simulink model "Controlled_SinglePhase_CenterTapde_Rectifier"  (R2021a)
settings: Solver=VariableStepAuto  StartTime=0.0  StopTime=0.1  MaxStep=1e-6  RelTol=1e-3
libraries: spsGroundLib x2, spsThyristorLib x2, spsVoltageMeasurementLib x2, spsACVoltageSourceLib x1, spsLinearTransformerLib x1, spsSeriesRLCBranchLib x1, spspowerguiLib x1
settings Model: Creator=mluser  LastModifiedBy=mluser

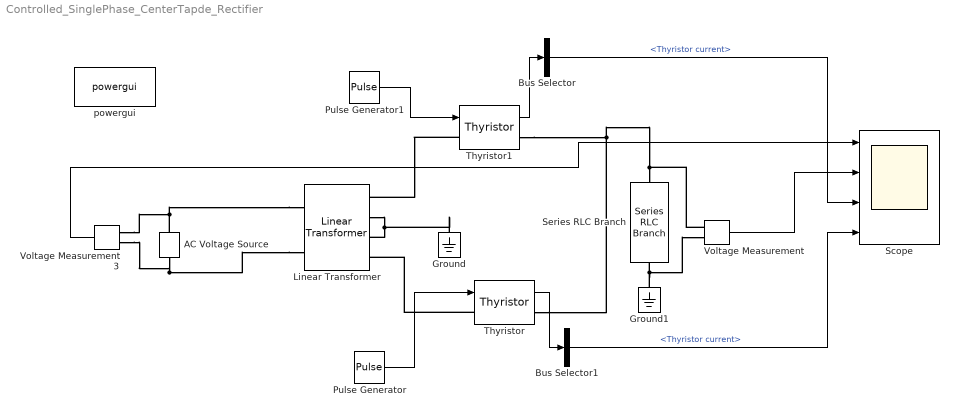
== system Controlled_SinglePhase_CenterTapde_Rectifier ==
  AC Voltage Source : spsACVoltageSourceLib/AC Voltage Source  Amplitude=30  Phase=0  Frequency=50  SampleTime=0  Measurements=None  BusType=swing  Pref=10e3  Qref=0  Qmin=-inf  Qmax=+inf
  Bus Selector : BusSelector  OutputSignals=Thyristor current
  Bus Selector1 : BusSelector  OutputSignals=Thyristor current
  Ground : spsGroundLib/Ground  LConnTagsString=a
  Ground1 : spsGroundLib/Ground  LConnTagsString=a
  Linear Transformer : spsLinearTransformerLib/Linear Transformer  UNITS=pu  NominalPower=[ 250e6 50 ]  winding1="[ 21.21  0.000  0.00 ]"  winding2="[ 21.21  0.000  0.00  ]"  ThreeWindings=on  winding3="[ 21.21  0.000  0.00 ]"  RmLm=[inf inf]  Measurements=None  DataType=off
  Pulse Generator : DiscretePulseGenerator  PulseType=Time based  Period=0.02  PulseWidth=50  PhaseDelay=((30+180)*0.02)/(360)
  Pulse Generator1 : DiscretePulseGenerator  PulseType=Time based  Period=0.02  PulseWidth=50  PhaseDelay=(30*0.02)/(360)
  Scope : Scope  NumInputPorts=4
  Series RLC Branch : spsSeriesRLCBranchLib/Series RLC Branch  LConnTagsString=__new0  RConnTagsString=__new0  BranchType=R  Resistance=10  Inductance=500e-3  SetiL0=off  InitialCurrent=0  Capacitance=1e-6  Setx0=off  InitialVoltage=0  Measurements=None
  Thyristor : spsThyristorLib/Thyristor  Ron=0.001  Lon=0  Vf=0.8  IC=0  Rs=500  Cs=250e-9  Measurements=on
  Thyristor1 : spsThyristorLib/Thyristor  Ron=0.001  Lon=0  Vf=0.8  IC=0  Rs=500  Cs=250e-9  Measurements=on
  Voltage Measurement : spsVoltageMeasurementLib/Voltage Measurement  PhasorSimulation=off  OutputType=Complex  PSBequivalent=0
  Voltage Measurement3 : spsVoltageMeasurementLib/Voltage Measurement  PhasorSimulation=off  OutputType=Complex  PSBequivalent=0
  powergui : spspowerguiLib/powergui  Priority=1  SimulationMode=Continuous  SampleTime=50e-6  frequency=60  Iterations=50  frequencyindice=50  Pbase=100e6  ErrMax=1e-4  UnitsV=kV  UnitsW=MW  buscounter=0  FunctionMessages=off  echomessages=off  EnableUseOfTLC=off  CurrentSourceSwitches=off  DisableSnubberDevices=off  DisableRonSwitches=off  DisableVfSwitches=off  DisplayEquations=off  AutomaticDiscreteSolvers=off  SolverType=Tustin/Backward Euler (TBE)  Interpol=off  ExternalGateDelay=off  methode=off  Ts=100  x0status=blocks  SPID=on  SwTol=0  HookPort=off  NonlinearTolerance=1e-4  nMaxIteration=100  ContinueOnMaxIteration=off  RestoreLinks=warning  ResistiveCurrentMeasurement=off  Frange=[0:2:500]  Ylog=off  Xlog=on  ShowGrid=off  save=off  variable=ZData  structure=0  ZoomFFT=off  StartTime=0.0  cycles=1  DisplayStyle=1  fundamental=60  FreqAxis=off  MaxFrequency=1000  frequencyindicesteady=1  RmsSteady=1  display=off
  wires:
  Voltage Measurement3/1 -> Scope/1
  Pulse Generator/1 -> Thyristor/1
  Pulse Generator1/1 -> Thyristor1/1
  Voltage Measurement/1 -> Scope/2
  Thyristor1/1 -> Bus Selector/1
  Thyristor/1 -> Bus Selector1/1
  Bus Selector/1 -> Scope/3  "<Thyristor current>"
  Bus Selector1/1 -> Scope/4  "<Thyristor current>"
  connections:
  Linear Transformer/RConn3 -- Linear Transformer/RConn2 -- Ground/LConn1
  Linear Transformer/LConn1 -- AC Voltage Source/RConn1 -- Voltage Measurement3/LConn1
  Series RLC Branch/RConn1 -- Ground1/LConn1 -- Voltage Measurement/LConn2
  Linear Transformer/LConn2 -- AC Voltage Source/LConn1 -- Voltage Measurement3/LConn2
  Thyristor1/LConn1 -- Linear Transformer/RConn1
  Thyristor/LConn1 -- Linear Transformer/RConn4
  Thyristor/RConn1 -- Voltage Measurement/LConn1 -- Series RLC Branch/LConn1 -- Thyristor1/RConn1
